simulink model "lab5_1_simulink"  (R2018a)
settings: Solver=VariableStepAuto  StartTime=0.0  StopTime=10.0  RelTol=1e-3
values from neighbouring files (symbols this model uses):
  a_0 = 1    [lab5_1.m]
  a_1 = 1    [lab5_1.m]
  a_2 = 1    [lab5_1.m]
  a_3 = 1    [lab5_1.m]
  b = 1    [lab5_1.m]    (also in lab5_2.m)
  x_1 = 0    [lab5_1.m]
  x_2 = 0    [lab5_1.m]
  x_3 = 0    [lab5_1.m]
settings Model: Creator=john  LastModifiedBy=john

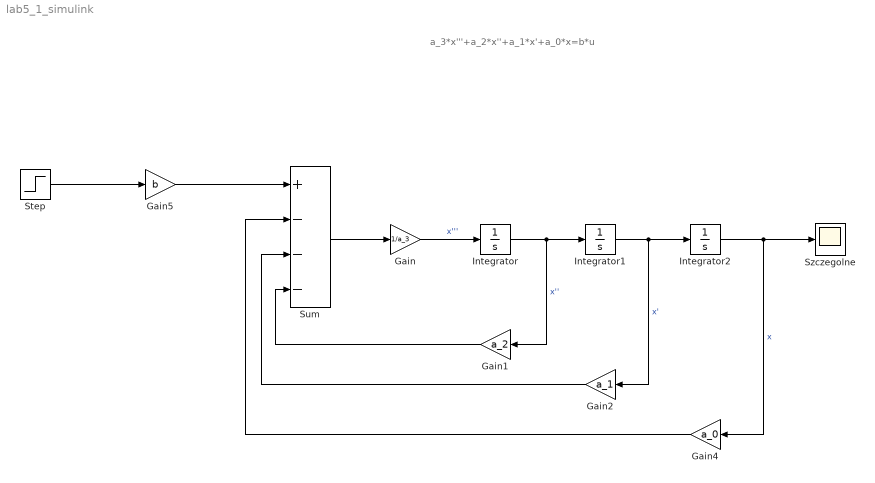
== system lab5_1_simulink ==
  note: a_3*x'''+a_2*x''+a_1*x'+a_0*x=b*u
  Gain : Gain  Gain=1/a_3
  Gain1 : Gain  Gain=a_2
  Gain2 : Gain  Gain=a_1
  Gain4 : Gain  Gain=a_0
  Gain5 : Gain  Gain=b
  Integrator : Integrator  InitialCondition=x_3
  Integrator1 : Integrator  InitialCondition=x_2
  Integrator2 : Integrator  InitialCondition=x_1
  Step : Step  SampleTime=0
  Sum : Sum  Inputs=+---
  "Szczegolne " : Scope
  wires:
  Integrator/1 -> Gain1/1, Integrator1/1  "x''"
  Integrator1/1 -> Gain2/1, Integrator2/1  "x'"
  Gain/1 -> Integrator/1  "x'''"
  Sum/1 -> Gain/1
  Integrator2/1 -> Gain4/1, "Szczegolne "/1  "x"
  Gain4/1 -> Sum/2
  Gain1/1 -> Sum/4
  Gain2/1 -> Sum/3
  Gain5/1 -> Sum/1
  Step/1 -> Gain5/1
